simulink model "S_function_Builder"  (R2024a)
settings: Solver=VariableStepAuto  StartTime=0.0  StopTime=10.0  RelTol=1e-3
model workspace (MAT data in the model file):
  configPath = Simulink.Parameter
  configPath.Complexity = 'real'
  configPath.Dimensions = [0 0]
  configPath.DataType = 'auto'
undefined symbols (not defined in the file or in its folder): aPath, readConfigFile
settings Model: Creator=deshazere  LastModifiedBy=deshazere

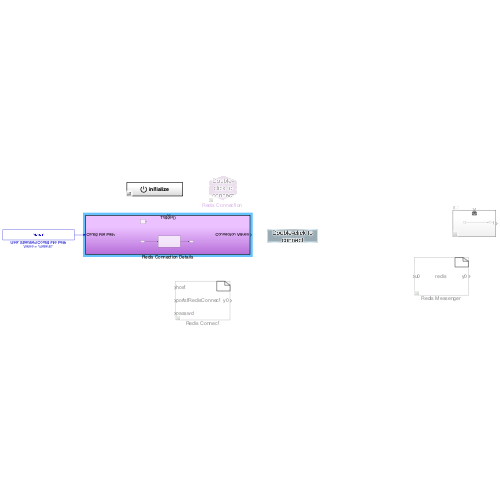
[thumbnail: Simulink's stored preview of the top-level diagram]
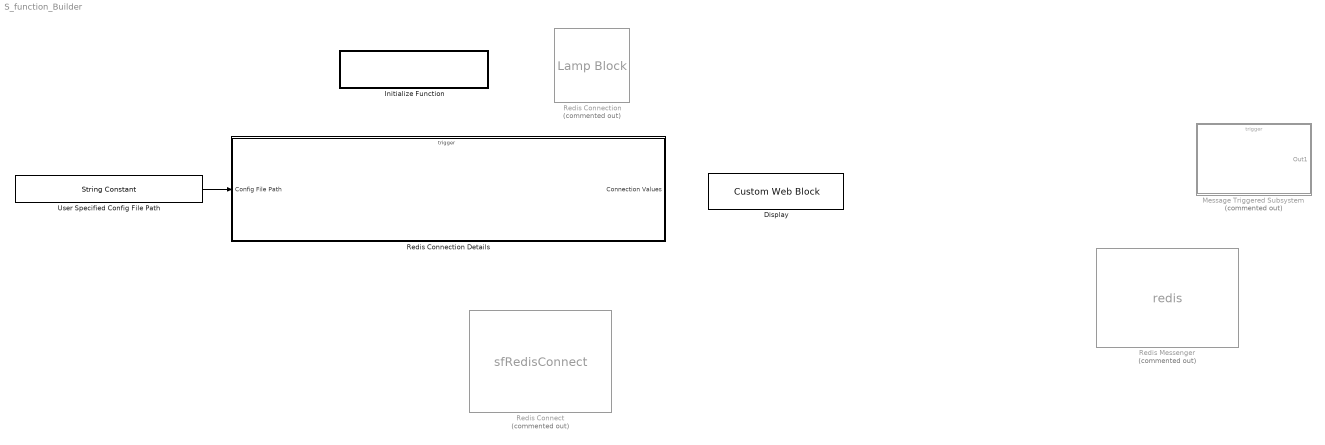
== system S_function_Builder ==
  Display : CustomWebBlock  LabelPosition=Hide  ShowInitialText=on  Configuration="{\"components\":[{\"name\":\"DisplayComponent\",\"settings\":{\"bold\":false,\"font\":\"DSEG7 Classic\",\"fontColor\":[255,255,200],\"fontSize\":\"14\",\"format\":\"short\",\"formatString\":\"%d\",\"italic\":false,\"position\":[1.22,0.22340425531914893,1,1],\"underline\":false}},{\"name\":\"BackgroundImageComponent\",\"settings\":{\"image\":{\"size\":[300,80],\"src\":\"data:image\\/svg+xml;base64,PHN2ZyBpZD0iZnJhbWUiIHhtbG5zPSJodHRwOi8vd3d3LnczLm9yZy8yMDAwL3N2ZyIgeG1sbnM6eGxpbms9Imh0dHA6Ly93d3cudzMub3JnLzE5OTkveGxpbmsiIHZpZXdCb3g9IjAgMCAzODAgMTAxIj48ZGVmcz48c3R5bGU+LmNscy0xe2ZpbGw6IzAwMmI0Mjt9LmNscy0ye2ZpbGw6IzQyNzA4Mjt9LmNscy0ze2ZpbGw6dXJsKCNyYWRpYWwtZ3JhZGllbnQpO308L3N0eWxlPjxyYWRpYWxHcmFkaWVudCBpZD0icmFkaWFsLWdyYWRpZW50IiBjeD0iMTkwIiBjeT0iNTAuNSIgcj0iMjY5LjIxIiBncmFkaWVudFVuaXRzPSJ1c2VyU3BhY2VPblVzZSI+PHN0b3Agb2Zmc2V0PSIwLjAxIiBzdG9wLWNvbG9yPSIjM2U0ZjU4Ii8+PHN0b3Agb2Zmc2V0PSIwLjA2IiBzdG9wLWNvbG9yPSIjNDQ1NzYxIi8+PHN0b3Agb2Zmc2V0PSIwLjE1IiBzdG9wLWNvbG9yPSIjNTU2YTc2Ii8+PHN0b3Agb2Zmc2V0PSIwLjI1IiBzdG9wLWNvbG9yPSIjNmQ4ODk1Ii8+PHN0b3Agb2Zmc2V0PSIwLjM4IiBzdG9wLWNvbG9yPSIjOGZiMmMzIi8+PHN0b3Agb2Zmc2V0PSIwLjUyIiBzdG9wLWNvbG9yPSIjYjZlNGZhIi8+PHN0b3Agb2Zmc2V0PSIxIiBzdG9wLWNvbG9yPSIjMTU0NjU3Ii8+PC9yYWRpYWxHcmFkaWVudD48L2RlZnM+PGcgaWQ9IkxheWVyXzIiIGRhdGEtbmFtZT0iTGF5ZXIgMiI+PGcgaWQ9IkxheWVyXzEtMiIgZGF0YS1uYW1lPSJMYXllciAxLTIiPjxyZWN0IGlkPSJyZWN0MTAzNiIgY2xhc3M9ImNscy0xIiB4PSIxMSIgeT0iMTEiIHdpZHRoPSIzNTgiIGhlaWdodD0iNzkiLz48cGF0aCBpZD0icGF0aDEwMzgiIGNsYXNzPSJjbHMtMiIgZD0iTTgsOFY5M0gzNzJWOFpNMzY5LDkwSDExVjExSDM2OVoiLz48cGF0aCBpZD0icGF0aDEwNDAiIGNsYXNzPSJjbHMtMyIgZD0iTTAsMFYxMDFIMzgwVjBaTTM3Miw5M0g4VjhIMzcyWiIvPjwvZz48L2c+PC9zdmc+\",\"srcOrientation\":\"Right\"},\"position\":[0,0,1,1],\"scaleMode\":\"0\"}},{\"name\":\"ForegroundImageComponent\",\"settings\":{\"angle\":0,\"image\":{\"size\":[0,0],\"src\":\"default\"},\"isForeground\":1,\"position\":[0,0,1,1],\"scaleMode\":\"0\"}}],\"settings\":{\"BindingType\":\"signal\",\"aspectRatio\":1.032258064516129,\"backgroundColor\":[0,0,0,\"1\"],\"backgroundOffset\":0.14,\"backgroundOpacity\":1,\"fixedAspectRatio\":\"on\",\"showBackgroundColor\":false,\"value\":0,\"version\":\"R2023b\"},\"type\":\"Display\"}"
  Initialize Function : Subsystem  InitFcn=readConfigFile  TreatAsAtomicUnit=on
  Message Triggered Subsystem : Subsystem  Commented=on  InputPortMessageModes=m  TreatAsAtomicUnit=on  ScheduleAs=Aperiodic partition  PartitionName=TEMP_PRECOMP_PARTITION_NAME_MessageTriggeredSubsystem
  Redis Connect : S-Function  Commented=on  FunctionName=sfRedisConnect  SFunctionModules=sfRedisConnect_wrapper.c  SFunctionDeploymentMode=off  EnableBusSupport=off  mask(S-Function Builder){}
      mask help: Simulink:masks:SFunctionBuilder_MD
      mask init:
      | val = [[.9  0.75 0.75 1 1 .9 .9 1]',[1 1 0.75 0.75 .9 .9 1 .9]'];try , sys = get_param(gcb,'SfunBuilderFcnName');if isempty(sys), sys = get_param(gcb,'FunctionName'); end,catch, sys = get_param(gcb,'FunctionName'); end
      settings: CopyFcn=set_param(gcbh,'LinkStatus','none')  OpenFcn=sfunctionwizard(gcbh)
      mask Display: plot(val(:,1),val(:,2)),disp(sys),port_label('input',1,'host'),port_label('input',2,'port'),port_label('input',3,'passwd'),port_label('output',1,'y0')
  Redis Connection : LampBlock  Commented=on  LabelPosition=Bottom  Icon=Custom  CustomIcon=data:image/svg+xml;base64,PCFET0NUWVBFIHN2ZyBQVUJMSUMgIi0vL1czQy8vRFREIFNWRyAxLjEvL0VOIiAiaHR0cDovL3d3dy53My5vcmcvR3JhcGhpY3MvU1ZHLzEuMS9EVEQvc3ZnMTEuZHRkIj4KPCEtLSBVcGxvYWRlZCB0bzogU1ZHIFJlcG8sIHd3dy5zdmdyZXBvLmNvbSwgVHJhbnNmb3JtZWQgYnk6IFNWRyBSZXBvIE1peGVyIFRvb2xzIC0tPgo8c3ZnIHdpZHRoPSI4MDBweCIgaGVpZ2h0PSI4MDBweCIgdmlld0JveD0iMCAtMTggMjU2IDI1NiIgeG1sbnM9Imh0dHA6Ly93d3cudzMub3JnLzIwMDAvc3ZnIiBwcmVzZXJ2ZUFzcGVjdFJhdGlvPSJ4 ...(+3816 chars)  Opacity=1.0
  Redis Connection Details : Subsystem  Priority=1  TreatAsAtomicUnit=on  ShowSubsystemReinitializePorts=on
      settings: AttributesFormatString=%<Description>
  Redis Messenger : S-Function  Commented=on  FunctionName=redis  SFunctionModules=redis_wrapper.c  SFunctionDeploymentMode=off  EnableBusSupport=off  mask(S-Function Builder){}
      mask help: Simulink:masks:SFunctionBuilder_MD
      mask init: same as S_function_Builder/Redis Connect
      settings: CopyFcn=set_param(gcbh,'LinkStatus','none')  OpenFcn=sfunctionwizard(gcbh)
      mask Display: plot(val(:,1),val(:,2)),disp(sys),port_label('input',1,'u0'),port_label('output',1,'y0')
  User Specified Config File Path : StringConstant  String="\"default\""
      settings: AttributesFormatString=Value = %<String>
  wires:
  User Specified Config File Path/1 -> Redis Connection Details/1(Config File Path)

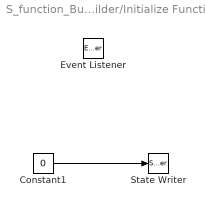
== system S_function_Builder/Initialize Function ==
  Constant1 : Constant  Value=0
  Event Listener : EventListener  DisableCoverage=on  EventName=reset  Variant=on
      settings: GeneratePreprocessorConditionals=on
  State Writer : StateWriter
  wires:
  Constant1/1 -> State Writer/1

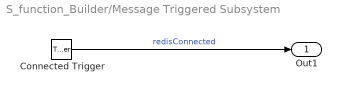
== system S_function_Builder/Message Triggered Subsystem ==
  Connected Trigger : TriggerPort  TriggerType=message  VariantControl=(inherit)  PortDimensions=1
  Out1 : Outport  InitialOutput=0
  wires:
  Connected Trigger/1 -> Out1/1  "redisConnected"

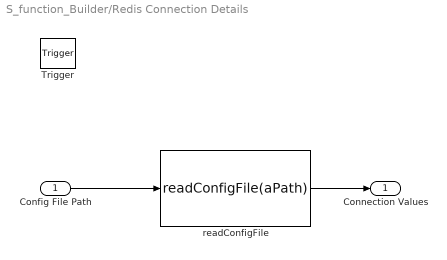
== system S_function_Builder/Redis Connection Details ==
  Config File Path : Inport
  Trigger : TriggerPort  TriggerType=function-call  VariantControl=(inherit)  ShowOutputPort=on  PortDimensions=1
  readConfigFile : MATLABFcn  Tag=Initialization  Description=|  Priority=1  MATLABFcn=readConfigFile(aPath)  OutputDimensions=3
      | Returns: host, port, and passwd
      | 
      | Args: alternative_redis_config_path
      | 
      | default:
      |     Mac/Linux: $HOME/.config/redis/irad_redis.config
      |     Windows:  $USERNAME/.config/redis/irad_redis.config
  Connection Values : Outport
  wires:
  Config File Path/1 -> readConfigFile/1
  readConfigFile/1 -> Connection Values/1
